simulink model "gstut7"  (Simulink 6.0)
settings: Solver=ode45  StartTime=0.0  StopTime=10.0  RelTol=1e-3
libraries: dspsrcs4 x2, dsparch4 x1, dspadpt3 x1
settings Model: LastModifiedBy=cclarke  UpdateModelReferenceTargets=IfOutOfDate
settings DataIOCC: SignalLoggingName=logsOut
settings DebuggingCC: CheckExecutionContextPreStartOutputMsg=on  CheckExecutionContextRuntimeOutputMsg=on
settings ModelReferenceCC: UpdateModelReferenceTargets=IfOutOfDate
settings GRTTargetCC: UtilityFuncGeneration=Automatic  LifeSpan=inf
settings SFSimCC: SFSimApplyToAllLibs=on  SFSimBuildMode=Incremental

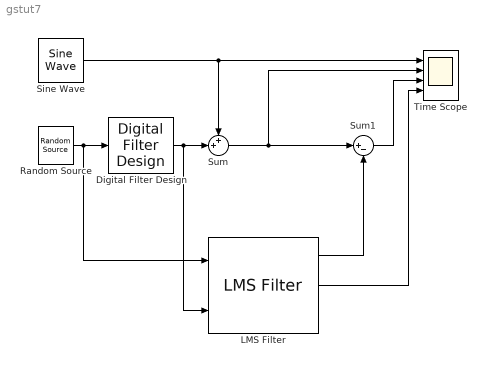
== system gstut7 ==
  Digital Filter Design : dsparch4/Digital Filter Design
  LMS Filter : dspadpt3/LMS Filter  DialogController=dspDDGCreate  DialogControllerArgs=DataTag1  Algo=Normalized LMS  L=32  stepflag=Dialog  mu=0.1  leakage=1.0  ic=0  Adapt=off  resetflag=None  weights=on  secondCoeffMode=User-defined  secondCoeffWordLength=2  secondCoeffFracLength=15  accum2Mode=User-defined  accum2FracLength=20  prodOutput2Mode=User-defined  prodOutput2FracLength=20  prodOutput3Mode=User-defined  prodOutput3FracLength=20  prodOutput4Mode=User-defined  prodOutput4FracLength=20  quotientMode=User-defined  quotientFracLength=20  roundingMode=Floor  overflowMode=off  addnparflag=off
  Random Source : dspsrcs4/Random Source  SrcType=Gaussian  NormMethod=Ziggurat  CltLength=12  Min=0  Max=1  Mean=0  Var=1  RepMode=Specify seed  rawSeed=[23341]  Inherit=off  SampMode=Discrete  SampTime=0.05  SampFrame=1  DataType=Double  OutComplex=Real
  Sine Wave : dspsrcs4/Sine Wave  Amplitude=1  Frequency=0.5  Phase=0  SampleMode=Discrete  OutComplex=Real  CompMethod=Trigonometric fcn  TableSize=Speed  SampleTime=0.05  SamplesPerFrame=1  dataType=double  wordLen=16  udDataType=sfix(16)  fracBitsMode=Best precision  numFracBits=15  ResetState=Restart at time zero
  Sum : Sum  Inputs=++|
  Sum1 : Sum  Inputs=|+-
  Time Scope : Scope  NumInputPorts=4
      settings: YMin=-5~-5~-5~-5  YMax=5~5~5~5  DataFormat=Structure
  wires:
  Sine Wave/1 -> Time Scope/1, Sum/1
  Random Source/1 -> Digital Filter Design/1, LMS Filter/1
  Sum/1 -> Time Scope/2, Sum1/1
  Digital Filter Design/1 -> Sum/2, LMS Filter/2
  LMS Filter/1 -> Sum1/2
  Sum1/1 -> Time Scope/3
  LMS Filter/2 -> Time Scope/4
